simulink model "lecture16_model"  (Simulink 7.6)
settings: Solver=ode45  StartTime=0.0  StopTime=10.0  RelTol=1e-3
values from neighbouring files (symbols this model uses):
  G1_den = [1 7 12]    [block_diagram_algrebra_example.m]
  G1_num = [3 -9]    [block_diagram_algrebra_example.m]
  G2_den = [1 26 197 408 720]    [block_diagram_algrebra_example.m]
  G2_num = [-2 -42 -142 -102]    [block_diagram_algrebra_example.m]
  H_den = [1 13 56 92 48]    [block_diagram_algrebra_example.m]
  H_num = [3 6 15]    [block_diagram_algrebra_example.m]
  T_den = [1 42 705 6176 31370 97888 195780 240192 142830]    [block_diagram_algrebra_example.m]
  T_num = [-2 -80 -1160 -7808 -25766 -40136 -25992 -4896]    [block_diagram_algrebra_example.m]
settings Model: Creator=lum  LastModifiedBy=lum
settings OptimizationCC: InitFltsAndDblsToZero=on
settings DebuggingCC: SaveWithParameterizedLinksMsg=none  StrictBusMsg=Warning
settings GRTTargetCC: TargetFcnLib=ansi_tfl_tmw.mat

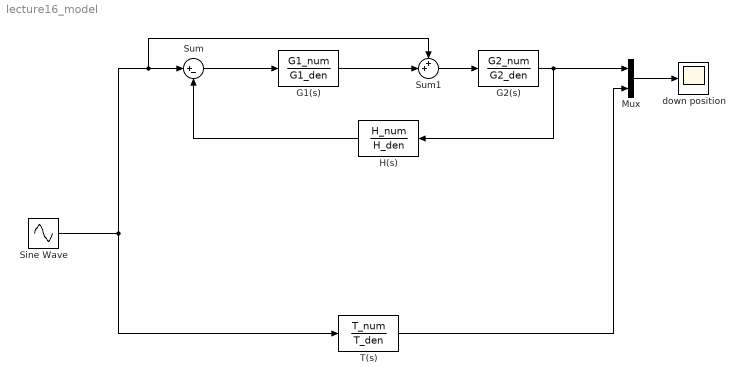
== system lecture16_model ==
  G1(s) : TransferFcn  Numerator=G1_num  Denominator=G1_den
  G2(s) : TransferFcn  Numerator=G2_num  Denominator=G2_den
  H(s) : TransferFcn  Numerator=H_num  Denominator=H_den
  Mux : Mux  Inputs=2
  Sine Wave : Sin  SampleTime=0
  Sum : Sum  Inputs=|+-
  Sum1 : Sum  Inputs=++|
  T(s) : TransferFcn  Numerator=T_num  Denominator=T_den
  down position : Scope
  wires:
  Mux/1 -> down position/1
  Sum/1 -> G1(s)/1
  G1(s)/1 -> Sum1/2
  Sum1/1 -> G2(s)/1
  G2(s)/1 -> H(s)/1, Mux/1
  Sine Wave/1 -> Sum/1, Sum1/1, T(s)/1
  H(s)/1 -> Sum/2
  T(s)/1 -> Mux/2
